simulink model "TurtleBotZeroDynamic"  (R2022b)
settings: Solver=FixedStepAuto  StartTime=0.0  StopTime=inf  RelTol=1e-3
StartFcn:
  | % Path del Blocco di cui vogliamo estrarre gli output
  | blk = 'TurtleBotZeroDynamic/Subscriber Odometria/Subsystem';
  | 
  | % Si allega al blocco in questione un event listener che esegue la funzione 'displayBusdata'
  | % in occasione dell'evento 'PostOutputs' ossia quando sono disponibili nuovi output dal blocco blk
  | h = add_exec_event_listener(blk, 'PostOutputs', @displayBusdata);
StopFcn:
  | pause(0.1);
  | if out.controllo_attivo.Data
  | 
  |      rng("shuffle");
  |      node_name = strcat("NODO_STOP_",num2str(randi([1000,9999])));
  |      fprintf("CREAZIONE %s\n",node_name);
  |      nodo = ros2node(node_name);
  | 
  |      pause(0.5)    % Permette la scrittura del segnale 'Scelta' nel workspace con il nome di 'scelta_turtlebot'
  | 
  |      if out.scelta_turtlebot.Data == 1
  |           disp('FERMO TURTLE 1')
  |           [pub, msg] = ros2publisher(nodo,'/turtle1/cmd_vel','geometry_msgs/Twist','Depth',1);
  |           %disp(pub)
  |       elseif out.scelta_turtlebot.Data == 2
  |           disp('FERMO TURTLE 2')
  |           [pub, msg] = ros2publisher(nodo,'/turtle2/cmd_vel','geometry_msgs/Twist','Depth',1);
  |           %disp(pub)
  |       elseif out.scelta_turtlebot.Data == 3
  |           disp('FERMO TURTLE 3')
  |           [pub, msg] = ros2publisher(nodo,'/turtle3/cmd_vel','geometry_msgs/Twist','Depth',1);
  |           %disp(pub)
  |      end
  | 
  |      %pause(1)
  | 
  |      send(pub,msg);
  | 
  |      pause(1);
  | 
  |      %delete(nodo);
  | 
  |  end
  | 
  |  % Do not delete, this is an auto-generated function to log ROS 2 message.
  |  ros.slros.internal.ROSUtil.logROSMessageToBagFile(bdroot);
  | 
  |  %clear all
  |  clear
model workspace (MAT data in the model file):
  ROSLoggingInfo_.GenBagFile = 1
  ROSLoggingInfo_.BagFileName = 'untitled'
  ROSLoggingInfo_.SerializationFormat = 'cdr'
  ROSLoggingInfo_.StorageFormat = 'sqlite3'
  ROSLoggingInfo_.CacheSize = 104857600
  ROSLoggingInfo_.LogOption = 'Default'
  ROSLoggingInfo_.FilePrefix = ''
  ROSLoggingReload_{1,1} = 'untitled/Subscribe'
  ROSLoggingReload_{2,1} = 'untitled/Blank Message'
  ROSLoggingReload_{3,1} = 'untitled/Bus
    | Assignment'
  ROSLoggingReload_{1,2} = 0
  ROSLoggingReload_{2,2} = 0
  ROSLoggingReload_{3,2} = 0
  ROSLoggingReload_{1,3} = 'my_topic_subscribe'
  ROSLoggingReload_{2,3} = 'blank_message'
  ROSLoggingReload_{3,3} = 'my_topic_bus_assignment'
  ROSLoggingTable_ = {}
  SL_ROS_VariableLengthArrays_MaxSizes.CommonInfo.ArrayTruncateAction = 'EmitWarning'
  SL_ROS_VariableLengthArrays_MaxSizes.MsgTypeMap = containers.Map
  SL_ROS_VariableLengthArrays_MaxSizes.MsgTypeMap.serialization.keys = {'std_msgs/Float32MultiArray', 'std_msgs/Float64MultiArray'}
  SL_ROS_VariableLengthArrays_MaxSizes.MsgTypeMap.serialization.values{1}.PropertyName = 'data'
  SL_ROS_VariableLengthArrays_MaxSizes.MsgTypeMap.serialization.values{1}.DataType = 'single'
  SL_ROS_VariableLengthArrays_MaxSizes.MsgTypeMap.serialization.values{1}.MaxLength = 2
  SL_ROS_VariableLengthArrays_MaxSizes.MsgTypeMap.serialization.values{2}.PropertyName = 'data'
  SL_ROS_VariableLengthArrays_MaxSizes.MsgTypeMap.serialization.values{2}.DataType = 'double'
  SL_ROS_VariableLengthArrays_MaxSizes.MsgTypeMap.serialization.values{2}.MaxLength = 3
  SL_ROS_VariableLengthArrays_MaxSizes.MsgTypeMap.serialization.uniformity = 0
  SL_ROS_VariableLengthArrays_MaxSizes.MsgTypeMap.serialization.keyType = 'char'
  SL_ROS_VariableLengthArrays_MaxSizes.MsgTypeMap.serialization.valueType = 'any'
undefined symbols (not defined in the file): angular, linear
libraries: ros2lib x10
(part 1 of 2)
PauseFcn:
  | % Istanza di un nodo ROS2
  | pause(0.1);
  | 
  | if out.controllo_attivo.Data
  | 
  |     rng("shuffle");
  |     node_name = strcat("NODO_PAUSE_",num2str(randi([1000,9999])));
  |     fprintf("CREAZIONE %s\n",node_name);
  |     nodo = ros2node(node_name);
  | 
  |      if out.scelta_turtlebot.Data == 1
  |           disp('PAUSA TURTLE 1')
  |           [pub, msg] = ros2publisher(nodo,'/turtle1/cmd_vel','geometry_msgs/Twist','Depth',1);
  |           %disp(pub)
  |       elseif out.scelta_turtlebot.Data == 2
  |           disp('PAUSA TURTLE 2')
  |           [pub, msg] = ros2publisher(nodo,'/turtle2/cmd_vel','geometry_msgs/Twist','Depth',1);
  |           %disp(pub)
  |       elseif out.scelta_turtlebot.Data == 3
  |           disp('PAUSA TURTLE 3')
  |           [pub, msg] = ros2publisher(nodo,'/turtle3/cmd_vel','geometry_msgs/Twist','Depth',1);
  |           %disp(pub)
  |      end
  | 
  |      pause(0.1)
  | 
  |      send(pub,msg);
  | 
  |      pause(0.01);
  | 
  |      delete(nodo);
  | 
  |      fprintf("CANCELLAZIONE %s\n",node_name);
  | 
  |  end
settings Model: Creator=Utente  LastModifiedBy=aless
settings OptimizationCC: EnhancedBackFolding=on  PassReuseOutputArgsAs=Individual arguments  ZeroExternalMemoryAtStartup=off  ZeroInternalMemoryAtStartup=off  MaxStackSize=64  OptimizeBlockOrder=speed  DifferentSizesBufferReuse=on  OptimizationCustomize=off  EfficientTunableParamExpr=on
settings DebuggingCC: ParameterTunabilityLossMsg=error
settings HardwareCC: UseEmbeddedCoderFeatures=off
settings SFSimCC: MATLABDynamicMemAlloc=off
settings RTWCC: Description=Embedded Coder  SystemTargetFile=ert.tlc  HardwareBoard=Robot Operating System 2 (ROS 2)  TLCOptions="-aInlineSetEventsForThisBaseRateFcn=TLC_FALSE -aSuppressMultiTaskScheduler=TLC_FALSE  -aRateBasedStepFcn=0"  TemplateMakefile=ert_default_tmf  Toolchain=Colcon Tools  TargetLang=C++
settings CodeAppCC: ForceParamTrailComments=on  IgnoreCustomStorageClasses=off  OperatorAnnotations=on  SimulinkDataObjDesc=on  SFDataObjDesc=on  InsertBlockDesc=on
settings ERTTargetCC: CodeInterfacePackaging=C++ class  SupportNonInlinedSFcns=on  RootIOFormat=Structure reference

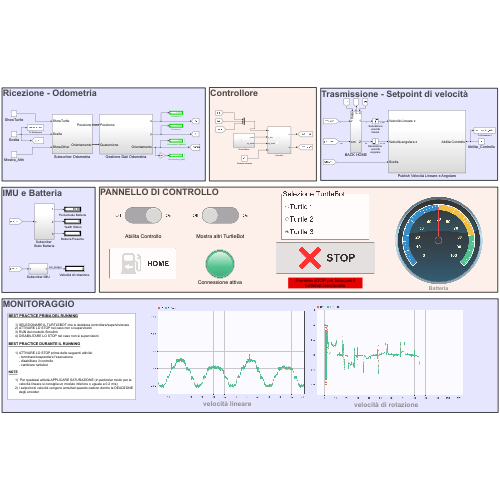
[thumbnail: Simulink's stored preview of the top-level diagram]
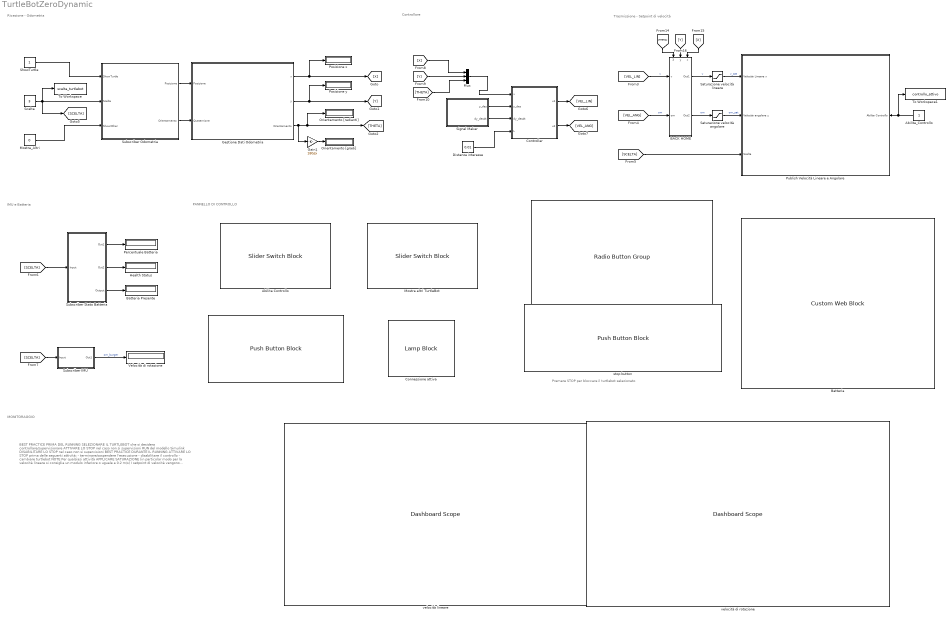
== system TurtleBotZeroDynamic ==
  note: BEST PRACTICE PRIMA DEL RUNNING
      |
      | SELEZIONARE IL TURTLEBOT che si desidera controllare/supervisionare
      | ATTIVARE LO STOP nel caso non si supervisioni
      | RUN del modello Simulink
      | DISABILITARE LO STOP nel caso non si supervisioni
      |
      | BEST PRACTICE DURANTE IL RUNNING
      |
      | ATTIVARE LO STOP prima delle seguenti attività:
      | - terminare/sospendere l'esecuzione
      | - disabilitare il controllo
      | - cambiare turtlebot
      |
      | NOTE
      |
      | Per qualsiasi attività APPLICARE SATURAZIONE (in particolar modo per la velocità lineare si consiglia un modulo inferiore o uguale a 0.2 m/s)
      | I setpoint di velocità vengono annullati quando cadono dentro la DEADZONE degli encoder
  note: MONITORAGGIO
  note: Controllore
  note: Trasmissione - Setpoint di velocità
  note: PANNELLO DI CONTROLLO
  note: IMU e Batteria
  note: Ricezione - Odometria
  note: Premere STOP per bloccare il turtlebot selezionato
  "  " : RadioButtonGroup  LabelPosition=Hide  SelectedLabel=Turtle 3  ButtonGroupName=Selezione TurtleBot
      settings: Values={{'Turtle 1', 'Turtle 2', 'Turtle 3'}, [1 2 3]}
  "    " : PushButtonBlock  ButtonText=HOME  ButtonType=Latch  Icon=Fuel  CustomIcon=data:image/png;base64,iVBORw0KGgoAAAANSUhEUgAAAgAAAAIACAYAAAD0eNT6AAAACXBIWXMAAA7DAAAOwwHHb6hkAAAAGXRFWHRTb2Z0d2FyZQB3d3cuaW5rc2NhcGUub3Jnm+48GgAAIABJREFUeJzt3Xm0p0V54PFvN9ANvbFJA4o2iwIKLiggAq7gghtiINFEMWrMTJIzmZPFJJMTHZMxBpPRSEwymUkmM6ImkzYq7oqKEVxwZWsUkM2NRWXphl7pvnf+qHtDo327772/qt9Tb9X3c85z4JgTfvU+71t166233ucFSZIkSZIkSZIkSZIkSZIkSZIkSZIkSZIkSZIkSZIkSZIkSZIkSZIkSZIkSZIkSZIkSZIkSZIkSZIkSZIkSZIkSZIkSZIkSZIkSZIkSZIkSZIk ...(+14436 chars)  IconColor=On  OffValue=0.000000
  Abilita Controllo : SliderSwitchBlock  LabelPosition=Hide
      settings: Values={{'Off', 'On'}, [2 1]}
  Abilita_Controllo : Constant  OutDataTypeStr=uint8
  BACK HOME : Subsystem
      settings: PortSchema="{\"entries\":[{\"content\":{\"sides\":[{\"content\":{\"connectorIds\":[\"In1\",\"In2\"]},\"type\":\"ConnectorPlacement.EquallySpacedRectSide\",\"uuid\":\"3e752b43-9c4b-4cec-95be-61bfbd83776f\"},{\"content\":{\"connectorIds\":[\"Out1\",\"Out2\"],\"side\":\"RIGHT\"},\"type\":\"ConnectorPlacement.EquallySpacedRectSide\",\"uuid\":\"e46021bd-fc58-40aa-a99c-da649cf669a0\"},{\"content\":{\"connectorIds\":[\"In3\",\"In4\",\"In5\"],\"side\":\"TOP\"},\"type\":\"ConnectorPlacement.EquallySpacedRectSide\",\"uuid\":\"6c89b280-edeb-4484-b9a1-ba484311f7be\"}]},\"type\":\"ConnectorPlacement.EquallySpacedConnector\",\"uuid\":\"6cd9684a-e5c4-4446-8d6f-4a7600db6ea4\"}],\"packageUris\":[\"http://schema.mathworks.com/mf0/Connector/R2020b\"],\"version\":\"1.0\"}"
  Batteria : CustomWebBlock  LabelPosition=Hide  ShowInitialText=on  Configuration="{\"components\":[{\"name\":\"CircularScaleComponent\",\"settings\":{\"bounds\":{\"max\":100,\"min\":0,\"tickInterval\":10},\"direction\":\"cw\",\"flipLimits\":0,\"innerRadius\":0.75,\"internalTickHeightScaleFactor\":1,\"labelColor\":[255,255,200],\"labelFont\":{\"font\":\"Arial\",\"fontSize\":12},\"labelRadius\":0.528,\"labelTransparency\":1,\"minorTickHeightScaleFactor\":0.2,\"needleImage\":{\"size\":[200,50],\"src\":\"data:image\\/svg+xml;base64,PD94bWwgdmVyc2lvbj0iMS4wIiBlbmNvZGluZz0idXRmLTgiPz4KPCEtLSBHZW5lcmF0b3I6IEFkb2JlIElsbHVzdHJhdG9yIDI0LjEuMiwgU1ZHIEV4cG9ydCBQbHVnLUluIC4gU1ZHIFZlcnNpb246IDYuMDAgQnVpbGQgMCkgIC0tPgo8c3ZnIHZlcnNpb249IjEuMSIgaWQ9IkxheWVyXzEiIHhtbG5zPSJodHRwOi8vd3d3LnczLm9yZy8yMDAwL3N2ZyIgeG1sbnM6eGxpbms9Imh0dHA6Ly93d3cudzMub3JnLzE5OTkveGxpbmsiIHg9IjBweCIgeT0iMHB4IgoJIHZpZXdCb3g9IjAgMCAyMDAgNTAiIHN0eWxlPSJlbmFibGUtYmFja2dyb3VuZDpuZXcgMCAwIDIwMCA1MDsiIHhtbDpzcGFjZT0icHJlc2VydmUiPgo8c3R5bGUgdHlwZT0idGV4dC9jc3MiPgoJLnN0MHtmaWxsOiNFQzIxMjc7fQo8L3N0eWxlPgo8cGF0aCBjbGFzcz0ic3QwIiBkPSJNMTYyLjgsMTMuN0MxNjksNC40LDE4MS43LDEuOSwxOTEsOC4xczExLjgsMTguOSw1LjYsMjguMnMtMTguOSwxMS44LTI4LjIsNS42bDAsMAoJQzE1OS4xLDM1LjYsMTU2LjYsMjMsMTYyLjgsMTMuN0wxNjIuOCwxMy43eiBNMTY1LjgsMTUuOGMtNS4xLDcuNi0zLjEsMTcuOSw0LjYsMjNjNy42LDUuMSwxNy45LDMuMSwyMy00LjYKCWM1LjEtNy42LDMuMS0xNy45LTQuNi0yM2wwLDBDMTgxLjIsNi4yLDE3MC45LDguMiwxNjUuOCwxNS44eiIvPgo8cGF0aCBjbGFzcz0ic3QwIiBkPSJNMC40LDI1Ljl2LTMuM2wxNTktMi41Yy0wLjcsMi42LTAuNyw1LjIsMCw3LjhMMC40LDI1Ljl6Ii8+CjxjaXJjbGUgY2xhc3M9InN0MCIgY3g9IjE3OS42IiBjeT0iMjQiIHI9IjAuNyIvPgo8L3N2Zz4K\"},\"needleOffset\":[0.18464878250906522,0],\"needleOrientation\":-45,\"needleRotation\":180,\"needleSize\":{\"height\":0.11741692305346914,\"width\":0.46108337545091255},\"outerRadius\":0.9,\"position\":[0.05,0.05,0.9,0.9],\"referencePoint\":\"auto\",\"scaleAngle\":270,\"scaleAngleOffset\":135,\"scaleColors\":[{\"Color\":[255,0,0],\"Max\":30,\"Min\":0},{\"Color\":[255,105,41],\"Max\":50,\"Min\":30},{\"Color\":[237,177,32],\"Max\":80,\"Min\":50},{\"Color\":[34,181,115],\"Max\":100,\"Min\":80}],\"scaleColorsSize\":0.2,\"scaleDirection\":\"CW\",\"scalePosition\":[0,0,1,1],\"showLabels\":1,\"showMinorTicks\":1,\"showSpanLine\":1,\"showTicks\":1,\"tickColor\":[255,255,255],\"tickTransparency\":1,\"valueBarColor\":[0,114,189],\"valueBarPosition\":[0,0,1,1],\"valueBarSize\":0.2,\"valueBarTransparency\":1}},{\"name\":\"BackgroundImageComponent\",\"settings\":{\"image\":{\"size\":[500,500],\"src\":\"data:image\\/svg+xml;base64,PD94bWwgdmVyc2lvbj0iMS4wIiBlbmNvZGluZz0iVVRGLTgiIHN0YW5kYWxvbmU9Im5vIj8+CjxzdmcKICAgeG1sbnM6ZGM9Imh0dHA6Ly9wdXJsLm9yZy9kYy9lbGVtZW50cy8xLjEvIgogICB4bWxuczpjYz0iaHR0cDovL2NyZWF0aXZlY29tbW9ucy5vcmcvbnMjIgogICB4bWxuczpyZGY9Imh0dHA6Ly93d3cudzMub3JnLzE5OTkvMDIvMjItcmRmLXN5bnRheC1ucyMiCiAgIHhtbG5zOnN2Zz0iaHR0cDovL3d3dy53My5vcmcvMjAwMC9zdmciCiAgIHhtbG5zPSJodHRwOi8vd3d3LnczLm9yZy8yMDAwL3N2ZyIKICAgeG1sbnM6 ...(+9964 chars)\"},\"position\":[0,0,1,1],\"scaleMode\":\"0\"}},{\"name\":\"ForegroundImageComponent\",\"settings\":{\"image\":{\"size\":[0,0],\"src\":\"default\",\"srcOrientation\":[]},\"isForeground\":1,\"position\":[0,0,1,1],\"scaleMode\":\"0\"}}],\"settings\":{\"BindingType\":\"signal\",\"aspectRatio\":1.032258064516129,\"backgroundColor\":[0,0,0,\"1\"],\"backgroundOffset\":1,\"backgroundOpacity\":1,\"direction\":\"cw\",\"fixedAspectRatio\":\"on\",\"flipLimits\":0,\"orientation\":\"horizontal\",\"showBackgroundColor\":false,\"value\":0,\"version\":\"R2022b\"},\"type\":\"CircularGauge\"}"
  Batteria Presente : Display
  Connessione attiva : LampBlock  LabelPosition=Hide
  Controller : Subsystem
  Distanza interasse : Constant  Value=0.01
  Gain1 : Gain  Gain=180/pi
  Gestione Dati Odometria : Subsystem
  Health Status : Display
  Mostra altri TurtleBot : SliderSwitchBlock  LabelPosition=Hide
      settings: Values={{'Off', 'On'}, [0 1]}
  Mostra_Altri : Constant  Value=0
  Mux : Mux  Inputs=3
  Orientamento [gradi] : Display
  Orientamento [radianti] : Display
  Percentuale Batteria : Display
  Posizione x : Display
  Posizione y : Display
  Publish Velocità Lineare e Angolare : Subsystem
      settings: PortSchema="{\"entries\":[{\"content\":{\"sides\":[{\"content\":{\"connectorIds\":[\"In1\",\"In2\",\"In3\"]},\"type\":\"ConnectorPlacement.EquallySpacedRectSide\",\"uuid\":\"492f9fe2-0066-41ae-950c-e30b37c64a5d\"},{\"content\":{\"connectorIds\":[\"In4\"],\"side\":\"RIGHT\"},\"type\":\"ConnectorPlacement.EquallySpacedRectSide\",\"uuid\":\"22b6dd94-4b9c-49f0-844e-1910cbdd2102\"},{\"content\":{\"side\":\"TOP\"},\"type\":\"ConnectorPlacement.EquallySpacedRectSide\",\"uuid\":\"8aae0b26-ff9a-4d56-9c5e-0be2d0f2fd36\"}]},\"type\":\"ConnectorPlacement.EquallySpacedConnector\",\"uuid\":\"44d0050b-2324-47f5-baee-e21b21bb071e\"}],\"packageUris\":[\"http://schema.mathworks.com/mf0/Connector/R2020b\"],\"version\":\"1.0\"}"
  Saturazione velocità lineare : Saturate  UpperLimit=0.1  LowerLimit=-0.1  LinearizeAsGain=off
  Saturazione velocità angolare : Saturate  UpperLimit=0.8  LowerLimit=-0.8  LinearizeAsGain=off
  Scelta : Constant  Value=3
  ShowTurtle : Constant  OutDataTypeStr=boolean
  Signal Maker : Subsystem
  Subscriber Stato Batteria : Subsystem
  Subscriber IMU : Subsystem
  Subscriber Odometria : Subsystem
  To Workspace : ToWorkspace  VariableName=scelta_turtlebot  SaveFormat=Timeseries  SampleTime=-1
      settings: MaxDataPoints=1
  To Workspace1 : ToWorkspace  VariableName=controllo_attivo  SaveFormat=Timeseries  SampleTime=-1
      settings: MaxDataPoints=1
  "Velocità di rotazione " : Display
  stop button : PushButtonBlock  ButtonText=STOP  ButtonType=Latch  Icon=Ex4  IconColor=On  OffValue=0.000000
  velocità di rotazione : DashboardScope  Ymin=-1  Ymax=1  UpdateMode=Scroll  NormalizeYAxis=on
  velocità lineare : DashboardScope  Ymin=-1  Ymax=1  UpdateMode=Scroll  NormalizeYAxis=on
  wires:
  Subscriber Stato Batteria/1(Out1) -> Percentuale Batteria/1
  Subscriber Stato Batteria/2(Out2) -> Health Status/1
  Subscriber IMU/1(Out1) -> "Velocità di rotazione "/1  "om_burger"
  Scelta/1 -> [SCELTA], Subscriber Odometria/2(Scelta), To Workspace/1
  Subscriber Odometria/1(Posizione) -> Gestione Dati Odometria/1(Posizione)
  Subscriber Odometria/2(Orientamento) -> Gestione Dati Odometria/2("Quaternione ")
  ShowTurtle/1 -> Subscriber Odometria/1(ShowTurtle)
  Gain1/1 -> Orientamento [gradi]/1
  Gestione Dati Odometria/3(Orientamento) -> [THETA], Orientamento [radianti]/1, Gain1/1
  Gestione Dati Odometria/2(y) -> [Y], Posizione y/1
  Gestione Dati Odometria/1(x) -> [X], Posizione x/1
  Abilita_Controllo/1 -> To Workspace1/1, Publish Velocità Lineare e Angolare/4(Abilita Controllo)
  Saturazione velocità angolare/1 -> Publish Velocità Lineare e Angolare/2(Velocità angolare z)  "om_sat"
  Saturazione velocità lineare/1 -> Publish Velocità Lineare e Angolare/1(Velocità Lineare x)  "v_sat"
  [SCELTA] -> Publish Velocità Lineare e Angolare/3(Scelta)
  [SCELTA] -> Subscriber Stato Batteria/1(Input)
  [SCELTA] -> Subscriber IMU/1(Input)
  Mostra_Altri/1 -> Subscriber Odometria/3(ShowOther)
  Subscriber Stato Batteria/3(Output) -> Batteria Presente/1
  [X] -> BACK HOME/5(x)
  [Y] -> BACK HOME/4(y)
  [THETA] -> BACK HOME/3(theta)
  [VEL_LIN] -> BACK HOME/1(v)  "v"
  [VEL_ANG] -> BACK HOME/2(om)  "om"
  BACK HOME/1(Out1) -> Saturazione velocità lineare/1  "v"
  BACK HOME/2(Out2) -> Saturazione velocità angolare/1  "om"
  Signal Maker/1(y_des) -> Controller/2(y_des)
  Signal Maker/2(dy_desdt) -> Controller/3(dy_desdt)
  Distanza interasse/1 -> Controller/4(L)
  [X] -> Mux/1
  [Y] -> Mux/2
  [THETA] -> Mux/3
  Mux/1 -> Controller/1(x)
  Controller/1(u1) -> [VEL_LIN]
  Controller/2(u2) -> [VEL_ANG]

== system TurtleBotZeroDynamic/BACK HOME ==
  v : Inport
  om : Inport  Port=2
  theta : Inport  Port=3
  y : Inport  Port=4
  x : Inport  Port=5
  Controllo HOME : Subsystem
  HOME : Constant  Value=0
  Switch : Switch  Criteria=u2 > Threshold  SaturateOnIntegerOverflow=off  InputSameDT=off
  Switch1 : Switch  Criteria=u2 > Threshold  SaturateOnIntegerOverflow=off  InputSameDT=off
  Out1 : Outport
  Out2 : Outport  Port=2
  wires:
  theta/1 -> Controllo HOME/3(theta)
  Controllo HOME/2(Velocità angolare) -> Switch1/1
  Controllo HOME/1(Velocità Lineare) -> Switch/1
  HOME/1 -> Controllo HOME/4(Input), Switch1/2, Switch/2
  om/1 -> Switch1/3
  y/1 -> Controllo HOME/2(y)
  v/1 -> Switch/3
  Switch1/1 -> Out2/1
  Switch/1 -> Out1/1
  x/1 -> Controllo HOME/1(x)

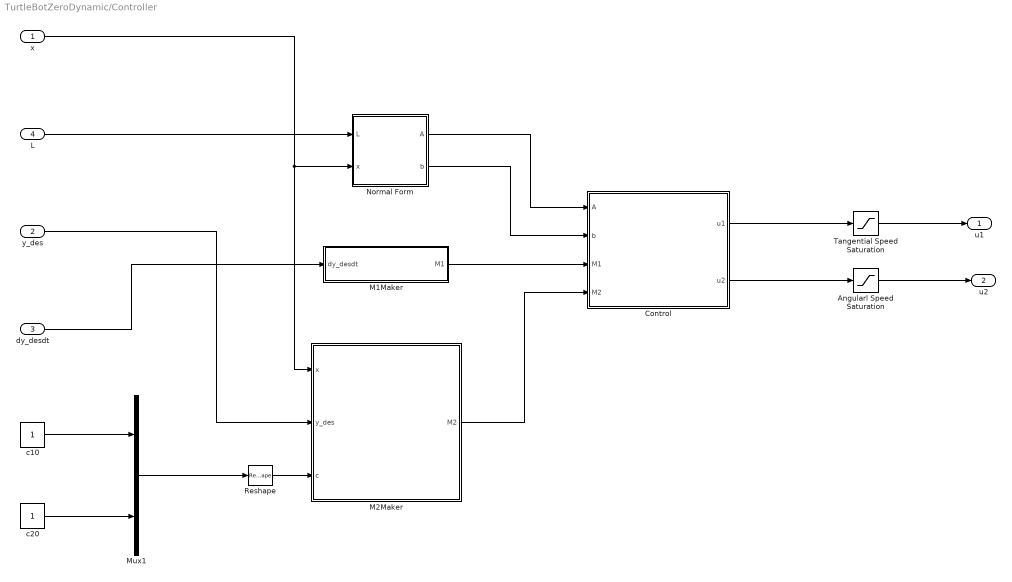
== system TurtleBotZeroDynamic/Controller ==
  x : Inport
  y_des : Inport  Port=2
  dy_desdt : Inport  Port=3
  L : Inport  Port=4
  Angularl Speed Saturation : Saturate  UpperLimit=1  LowerLimit=-1
  Control : MATLAB Function  TreatAsAtomicUnit=on
  M1Maker : Subsystem
  M2Maker : MATLAB Function  TreatAsAtomicUnit=on
  Mux1 : Mux  Inputs=2
  Normal Form : MATLAB Function  TreatAsAtomicUnit=on
  Reshape : Reshape  OutputDimensionality=Column vector (2-D)
  Tangential Speed Saturation : Saturate  UpperLimit=0.15  LowerLimit=-0.15
  c10 : Constant
  c20 : Constant
  u1 : Outport
  u2 : Outport  Port=2
  wires:
  y_des/1 -> M2Maker/2(y_des)
  Normal Form/1(A) -> Control/1(A)
  M1Maker/1(M1) -> Control/3(M1)
  x/1 -> Normal Form/2(x), M2Maker/1(x)
  Normal Form/2(b) -> Control/2(b)
  M2Maker/1(M2) -> Control/4(M2)
  Mux1/1 -> Reshape/1
  c10/1 -> Mux1/1
  Reshape/1 -> M2Maker/3(c)
  Control/1(u1) -> Tangential Speed Saturation/1
  c20/1 -> Mux1/2
  dy_desdt/1 -> M1Maker/1(dy_desdt)
  L/1 -> Normal Form/1(L)
  Control/2(u2) -> Angularl Speed Saturation/1
  Tangential Speed Saturation/1 -> u1/1
  Angularl Speed Saturation/1 -> u2/1

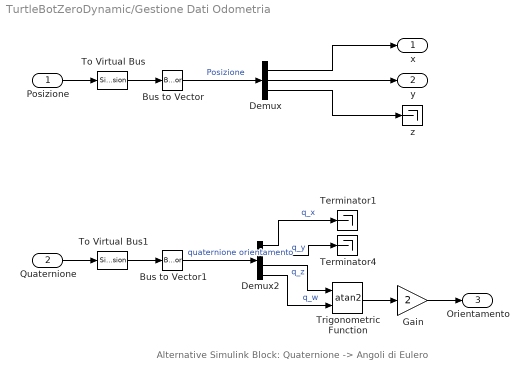
== system TurtleBotZeroDynamic/Gestione Dati Odometria ==
  note: Alternative Simulink Block: Quaternione -> Angoli di Eulero
  Posizione : Inport
  "Quaternione " : Inport  Port=2
  Bus to Vector : BusToVector
  Bus to Vector1 : BusToVector
  Demux : Demux  Outputs=3
  Demux2 : Demux
  Gain : Gain  Gain=2
  Terminator1 : Terminator
  Terminator4 : Terminator
  To Virtual Bus : SignalConversion  ConversionOutput=Virtual bus  OverrideOpt=off
  To Virtual Bus1 : SignalConversion  ConversionOutput=Virtual bus  OverrideOpt=off
  Trigonometric Function : Trigonometry  Operator=atan2
  z : Terminator
  x : Outport
  y : Outport  Port=2
  Orientamento : Outport  Port=3
  wires:
  Demux2/1 -> Terminator1/1  "q_x"
  "Quaternione "/1 -> To Virtual Bus1/1
  Bus to Vector1/1 -> Demux2/1  "quaternione orientamento"
  Demux2/2 -> Terminator4/1  "q_y"
  To Virtual Bus/1 -> Bus to Vector/1
  Demux/3 -> z/1
  Bus to Vector/1 -> Demux/1  "Posizione"
  Gain/1 -> Orientamento/1
  Trigonometric Function/1 -> Gain/1
  Demux2/4 -> Trigonometric Function/2  "q_w"
  Demux/1 -> x/1
  To Virtual Bus1/1 -> Bus to Vector1/1
  Demux2/3 -> Trigonometric Function/1  "q_z"
  Posizione/1 -> To Virtual Bus/1
  Demux/2 -> y/1

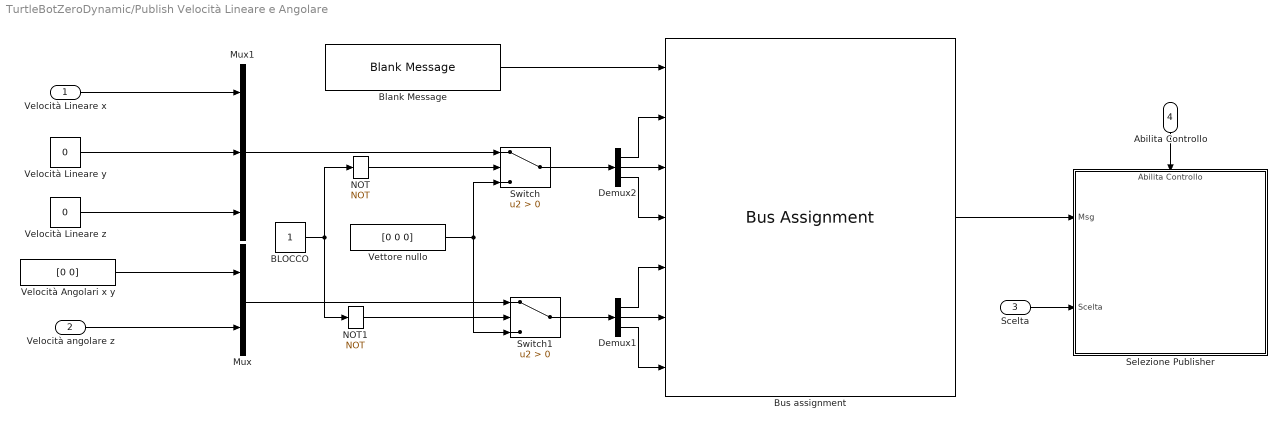
== system TurtleBotZeroDynamic/Publish Velocità Lineare e Angolare ==
  Velocità Lineare x : Inport
  Velocità angolare z : Inport  Port=2
  Scelta : Inport  Port=3
  Abilita Controllo : Inport  Port=4
  BLOCCO : Constant  OutDataTypeStr=boolean  SampleTime=-1  LockScale=on
  Blank Message : ros2lib/Blank Message  messageClass=Message  entityType=geometry_msgs/Twist  messageType=geometry_msgs/Twist  SampleTime=0.01
  Bus assignment : BusAssignment  AssignedSignals=linear.x,linear.y,linear.z,angular.x,angular.y,angular.z
  Demux1 : Demux  Outputs=3
  Demux2 : Demux  Outputs=3
  Mux : Mux  Inputs=2
  Mux1 : Mux  Inputs=3
  NOT : Logic  Operator=NOT  IconShape=distinctive  AllPortsSameDT=off  OutDataTypeStr=boolean
  NOT1 : Logic  Operator=NOT  IconShape=distinctive  AllPortsSameDT=off  OutDataTypeStr=boolean
  Selezione Publisher : Subsystem
      settings: PortSchema="{\"entries\":[{\"content\":{\"sides\":[{\"content\":{\"connectorIds\":[\"In1\",\"In2\"]},\"type\":\"ConnectorPlacement.EquallySpacedRectSide\",\"uuid\":\"6bd875f6-5ae5-4f8d-a0e5-50c836e94d9a\"},{\"content\":{\"side\":\"RIGHT\"},\"type\":\"ConnectorPlacement.EquallySpacedRectSide\",\"uuid\":\"9a720333-0721-45e1-af7e-2ea4384a1b06\"},{\"content\":{\"connectorIds\":[\"In3\"],\"side\":\"TOP\"},\"type\":\"ConnectorPlacement.EquallySpacedRectSide\",\"uuid\":\"e7c848f8-6ead-4da8-abb2-d4d43fa7a51b\"}]},\"type\":\"ConnectorPlacement.EquallySpacedConnector\",\"uuid\":\"46f07b8a-e3bc-456b-915d-31c6a07cabd2\"}],\"packageUris\":[\"http://schema.mathworks.com/mf0/Connector/R2020b\"],\"version\":\"1.0\"}"
  Switch : Switch  Criteria=u2 > Threshold  SaturateOnIntegerOverflow=off  InputSameDT=off
  Switch1 : Switch  Criteria=u2 > Threshold  SaturateOnIntegerOverflow=off  InputSameDT=off
  Velocità Angolari x y : Constant  Value=[0 0]  SampleTime=-1
  Velocità Lineare y : Constant  Value=0  SampleTime=-1
  Velocità Lineare z : Constant  Value=0  SampleTime=-1
  Vettore nullo : Constant  Value=[0 0 0]  SampleTime=-1
  wires:
  Demux2/2 -> Bus assignment/3
  Demux1/3 -> Bus assignment/7
  Vettore nullo/1 -> Switch1/3, Switch/3
  Demux1/2 -> Bus assignment/6
  Demux2/3 -> Bus assignment/4
  Demux1/1 -> Bus assignment/5
  BLOCCO/1 -> NOT1/1, NOT/1
  Switch/1 -> Demux2/1
  Demux2/1 -> Bus assignment/2
  Switch1/1 -> Demux1/1
  Mux/1 -> Switch1/1
  Velocità Angolari x y/1 -> Mux/1
  Velocità angolare z/1 -> Mux/2
  Velocità Lineare x/1 -> Mux1/1
  Mux1/1 -> Switch/1
  Velocità Lineare y/1 -> Mux1/2
  Blank Message/1 -> Bus assignment/1
  Velocità Lineare z/1 -> Mux1/3
  Scelta/1 -> Selezione Publisher/2(Scelta)
  Bus assignment/1 -> Selezione Publisher/1(Msg)
  Abilita Controllo/1 -> Selezione Publisher/3(Abilita Controllo)
  NOT/1 -> Switch/2
  NOT1/1 -> Switch1/2

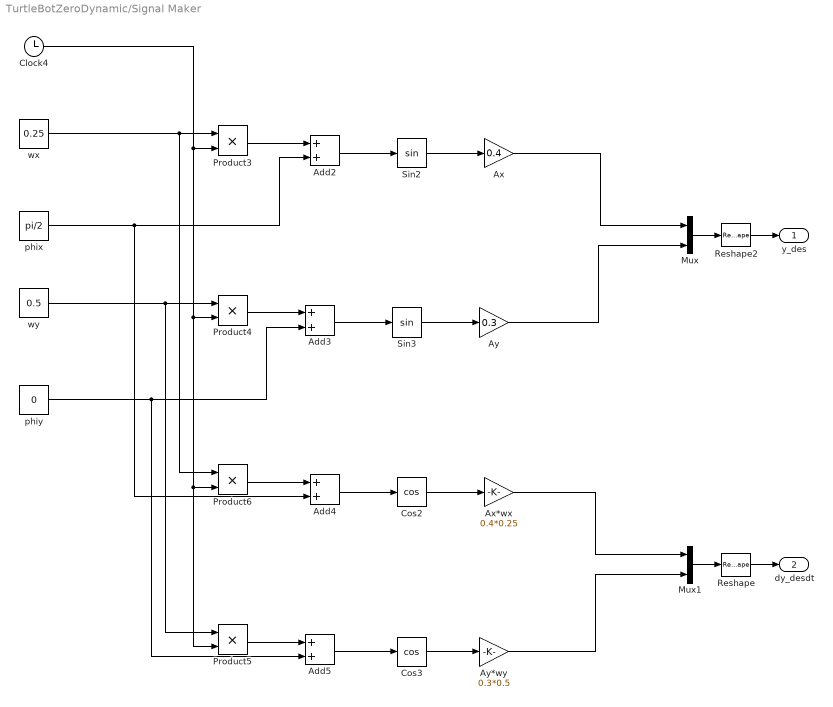
== system TurtleBotZeroDynamic/Signal Maker ==
  Add{2..5} (4 alike) : Sum
  Ax : Gain  Gain=0.4
  Ax*wx : Gain  Gain=0.4*0.25
  Ay : Gain  Gain=0.3
  Ay*wy : Gain  Gain=0.3*0.5
  Clock4 : Clock
  Cos2 : Trigonometry  Operator=cos
  Cos3 : Trigonometry  Operator=cos
  Mux : Mux  Inputs=2
  Mux1 : Mux  Inputs=2
  Product{3..6} (4 alike) : Product
  Reshape : Reshape  OutputDimensionality=Column vector (2-D)
  Reshape2 : Reshape  OutputDimensionality=Column vector (2-D)
  Sin2 : Trigonometry
  Sin3 : Trigonometry
  phix : Constant  Value=pi/2
  phiy : Constant  Value=0
  wx : Constant  Value=0.25
  wy : Constant  Value=0.5
  y_des : Outport
  dy_desdt : Outport  Port=2
  wires:
  Ax/1 -> Mux/1
  Reshape2/1 -> y_des/1
  Ay*wy/1 -> Mux1/2
  Product6/1 -> Add4/1
  Add4/1 -> Cos2/1
  Mux1/1 -> Reshape/1
  Add5/1 -> Cos3/1
  Product4/1 -> Add3/1
  wy/1 -> Product5/1, Product4/1
  phix/1 -> Add4/2, Add2/2
  Clock4/1 -> Product5/2, Product6/2, Product4/2, Product3/2
  Add2/1 -> Sin2/1
  Ax*wx/1 -> Mux1/1
  Sin2/1 -> Ax/1
  Ay/1 -> Mux/2
  Product3/1 -> Add2/1
  Cos2/1 -> Ax*wx/1
  wx/1 -> Product6/1, Product3/1
  Add3/1 -> Sin3/1
  phiy/1 -> Add5/2, Add3/2
  ? -> ?
  ? -> ?
  Sin3/1 -> Ay/1
  Reshape/1 -> dy_desdt/1
  Product5/1 -> Add5/1
  Cos3/1 -> Ay*wy/1
  Mux/1 -> Reshape2/1

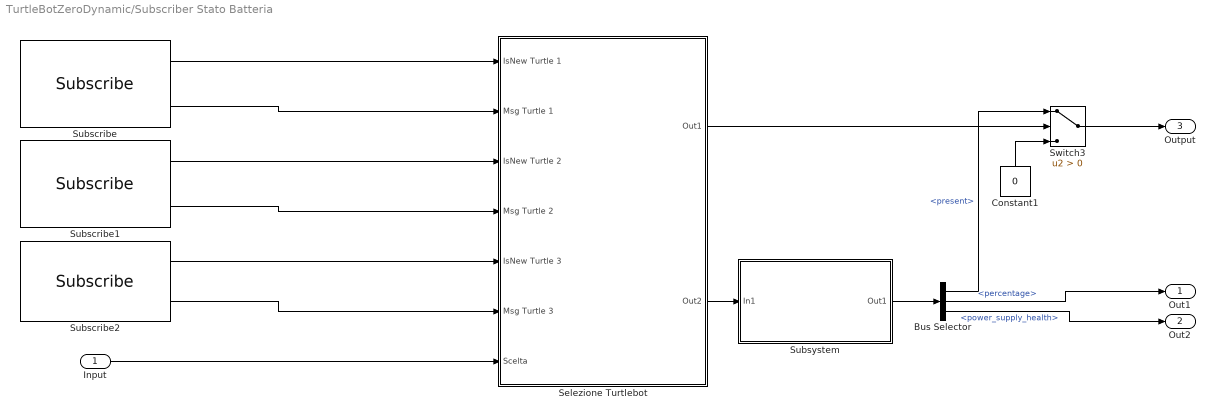
== system TurtleBotZeroDynamic/Subscriber Stato Batteria ==
  Input : Inport
  Bus Selector : BusSelector  OutputSignals=present,percentage,power_supply_health
  Constant1 : Constant  Value=0
  Selezione Turtlebot : Subsystem
  Subscribe : ros2lib/Subscribe  topicSource=Specify your own  topic=/turtle1/battery_state  messageType=sensor_msgs/BatteryState  sampleTime=1  QOSHistory=Keep last  QOSDepth=1  QOSReliability=Reliable  QOSDurability=Volatile
  Subscribe1 : ros2lib/Subscribe  topicSource=Specify your own  topic=/turtle2/battery_state  messageType=sensor_msgs/BatteryState  sampleTime=1  QOSHistory=Keep last  QOSDepth=1  QOSReliability=Reliable  QOSDurability=Volatile
  Subscribe2 : ros2lib/Subscribe  topicSource=Specify your own  topic=/turtle3/battery_state  messageType=sensor_msgs/BatteryState  sampleTime=1  QOSHistory=Keep last  QOSDepth=1  QOSReliability=Reliable  QOSDurability=Volatile
  Subsystem : Subsystem
  Switch3 : Switch  Criteria=u2 > Threshold  SaturateOnIntegerOverflow=off  InputSameDT=off
  Out1 : Outport
  Out2 : Outport  Port=2
  Output : Outport  Port=3
  wires:
  Subsystem/1(Out1) -> Bus Selector/1
  Bus Selector/2 -> Out1/1  "<percentage>"
  Bus Selector/3 -> Out2/1  "<power_supply_health>"
  Selezione Turtlebot/2(Out2) -> Subsystem/1(In1)
  Subscribe/1 -> Selezione Turtlebot/1(IsNew Turtle 1)
  Subscribe/2 -> Selezione Turtlebot/2(Msg Turtle 1)
  Subscribe1/1 -> Selezione Turtlebot/3(IsNew Turtle 2)
  Subscribe1/2 -> Selezione Turtlebot/4(Msg Turtle 2)
  Input/1 -> Selezione Turtlebot/7(Scelta)
  Subscribe2/2 -> Selezione Turtlebot/6(Msg Turtle 3)
  Subscribe2/1 -> Selezione Turtlebot/5(IsNew Turtle 3)
  Selezione Turtlebot/1(Out1) -> Switch3/2
  Switch3/1 -> Output/1
  Bus Selector/1 -> Switch3/1  "<present>"
  Constant1/1 -> Switch3/3

== system TurtleBotZeroDynamic/Subscriber IMU ==
  Input : Inport
  Bus Selector : BusSelector  OutputSignals=angular_velocity.z
  Selezione Turtlebot : Subsystem
  Subscribe : ros2lib/Subscribe  topicSource=Specify your own  topic=/turtle1/imu  messageType=sensor_msgs/Imu  sampleTime=0.05  QOSHistory=Keep last  QOSDepth=1  QOSReliability=Reliable  QOSDurability=Volatile
  Subscribe1 : ros2lib/Subscribe  topicSource=Specify your own  topic=/turtle2/imu  messageType=sensor_msgs/Imu  sampleTime=0.05  QOSHistory=Keep last  QOSDepth=1  QOSReliability=Reliable  QOSDurability=Volatile
  Subscribe2 : ros2lib/Subscribe  topicSource=Specify your own  topic=/turtle3/imu  messageType=sensor_msgs/Imu  sampleTime=0.05  QOSHistory=Keep last  QOSDepth=1  QOSReliability=Reliable  QOSDurability=Volatile
  Subsystem : Subsystem
  Out1 : Outport
  wires:
  Subsystem/1(Out1) -> Bus Selector/1
  Bus Selector/1 -> Out1/1  "<z>"
  Selezione Turtlebot/2(Out2) -> Subsystem/1(In1)
  Selezione Turtlebot/1(Out1) -> Subsystem/Enable
  Subscribe/1 -> Selezione Turtlebot/1(IsNew Turtle 1)
  Subscribe/2 -> Selezione Turtlebot/2(Msg Turtle 1)
  Subscribe1/1 -> Selezione Turtlebot/3(IsNew Turtle 2)
  Subscribe1/2 -> Selezione Turtlebot/4(Msg Turtle 2)
  Subscribe2/1 -> Selezione Turtlebot/5(IsNew Turtle 3)
  Subscribe2/2 -> Selezione Turtlebot/6(Msg Turtle 3)
  Input/1 -> Selezione Turtlebot/7(Scelta)
